simulink model "car10_23"  (Simulink 8.7)
settings: Solver=ode3  StartTime=0.0  StopTime=100  FixedStep=0.000250  RelTol=1e-3
libraries: Solver_SF x1, dspnetwork x1
settings Model: Creator=xuwei  LastModifiedBy=14755
settings DataIOCC: SaveFormat=StructureWithTime  SignalLoggingSaveFormat=ModelDataLogs
settings OptimizationCC: BlockReduction=off  OptimizeBlockIOStorage=off  BufferReuse=off  GlobalBufferReuse=off  ExpressionFolding=off  ExpressionDepthLimit=2147483647  LocalBlockOutputs=off
settings DebuggingCC: SolverPrmCheckMsg=warning  FcnCallInpInsideContextMsg=EnableAllAsWarning  StateNameClashWarn=warning
settings HardwareCC: ProdIntDivRoundTo=Zero  ProdEndianess=LittleEndian  ProdLongLongMode=on  ProdHWDeviceType=Generic->32-bit x86 compatible
settings RTWCC: CodeExecutionProfiling=on  RTWCompilerOptimization=on
settings CodeAppCC: MaxIdLength=95
settings GRTTargetCC: GeneratePreprocessorConditionals=Use local settings
settings ConfigComp: CovModelRefEnable=off

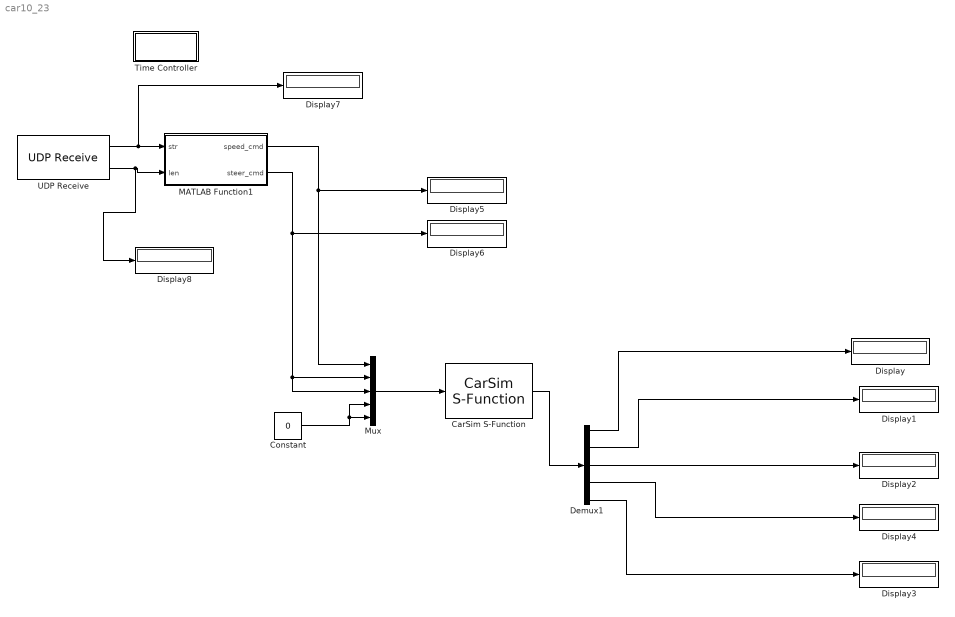
== system car10_23 ==
  CarSim S-Function : Solver_SF/CarSim S-Function  Priority=1  VehicleCode=i_i  SIMFILE=simfile.sim
  Constant : Constant  Value=0
  Demux1 : Demux  Outputs=5
  Display{,1..8} (9 alike) : Display
  MATLAB Function1 : MATLAB Function  TreatAsAtomicUnit=on
  Mux : Mux  Inputs=5
  Time Controller : Subsystem  mask(CarSim DS){}
      mask help: This Real-Time control block enables the Simulink system running at real time mode.
      mask init:
      | TimeStep=str2num(get_param(gcs,'FixedStep'));
      mask Display: disp('RT Enable');
  UDP Receive : dspnetwork/UDP Receive  localURL='0.0.0.0'  localPort=8887  remoteURL='0.0.0.0'  remotePort=-1  recvBufferSize=8192  dims=3  signalDatatype=double  isVarSize=off  showBlockingTime=off  blockingTime=0  sampletime=0.001
  wires:
  CarSim S-Function/1 -> Demux1/1
  Mux/1 -> CarSim S-Function/1
  Demux1/1 -> Display/1
  Demux1/2 -> Display1/1
  Demux1/3 -> Display2/1
  Demux1/4 -> Display4/1
  Demux1/5 -> Display3/1
  Constant/1 -> Mux/4, Mux/5
  MATLAB Function1/1(speed_cmd) -> Display5/1, Mux/1
  MATLAB Function1/2(steer_cmd) -> Mux/3, Mux/2, Display6/1
  UDP Receive/1 -> Display7/1, MATLAB Function1/1(str)
  UDP Receive/2 -> Display8/1, MATLAB Function1/2(len)

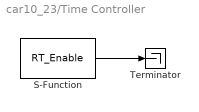
== system car10_23/Time Controller ==
  S-Function : S-Function  FunctionName=RT_Enable  Parameters=TimeStep  SFunctionDeploymentMode=off  EnableBusSupport=off
  Terminator : Terminator
  wires:
  S-Function/1 -> Terminator/1

== matlab function MATLAB Function1 ==
  data: str input double; speed_cmd output double; steer_cmd output double; len input double
function [speed_cmd,steer_cmd] = fcn(str, len)
persistent wait_flag;
persistent steer;
persistent speed;
if isempty(steer)
    steer=0;
end
if isempty(speed)
    speed=0;
end
if(len>0)
    speed = double(str(1));
    
    steer = double(str(3));
    wait_flag = 0;
end
% if isempty(wait_flag)
%     pause(5);
% end

steer_cmd = double(steer);
speed_cmd = double(speed);

%[speed_cmd,steer_cmd] = comunicate(x,y,yaw,vx,steer);
%00 00 00 00 00 00 24 40 00 00 00 00 00 00 00 00 00 00 00 00 00 00 00 00
